simulink model "Simulink_7"  (R2013b)
settings: Solver=FixedStepDiscrete  StartTime=0.0  StopTime=100.0  FixedStep=1  RelTol=1e-3
undefined symbols (not defined in the file or in its folder): j, magnitude
settings Model: ExtModeAutoUpdateStatusClock=off  Creator=asteele  LastModifiedBy=99900361
settings DataIOCC: SignalLoggingSaveFormat=ModelDataLogs  SignalLoggingName=sigsOut
settings OptimizationCC: BooleanDataType=off
settings DebuggingCC: SaveWithParameterizedLinksMsg=none  SignalResolutionControl=TryResolveAllWithWarning  SolverPrmCheckMsg=none  MultiTaskDSMMsg=warning  MultiTaskCondExecSysMsg=none  StrictBusMsg=None
settings HardwareCC: TargetUnknown=on
settings RTWCC: IncludeERTFirstTime=on
settings GRTTargetCC: CombineOutputUpdateFcns=off  GRTInterface=on

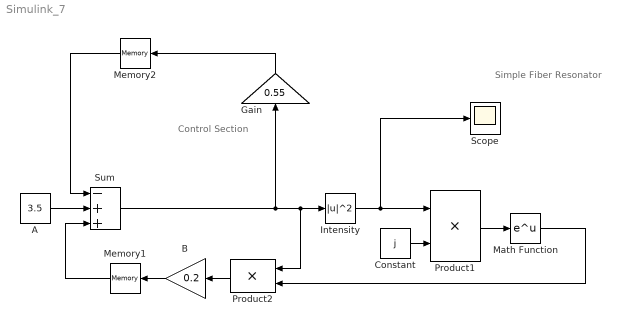
== system Simulink_7 ==
  note: Control Section
  note: Simple Fiber Resonator
  A : Constant  Value=3.5
  B : Gain  Gain=0.2  SaturateOnIntegerOverflow=on  OutDataTypeStr=Inherit: Same as input  ParamDataTypeStr=Inherit: Same as input
  Constant : Constant  Value=j
  Gain : Gain  Gain=0.55  SaturateOnIntegerOverflow=on  OutDataTypeStr=Inherit: Same as input  ParamDataTypeStr=Inherit: Same as input
  Intensity : Math  Operator=magnitude^2  SaturateOnIntegerOverflow=on
  Math Function : Math  SaturateOnIntegerOverflow=on
  Memory1 : Memory
  Memory2 : Memory
  Product1 : Product  SaturateOnIntegerOverflow=on  InputSameDT=on  OutDataTypeStr=Inherit: Same as first input
  Product2 : Product  SaturateOnIntegerOverflow=on  InputSameDT=on  OutDataTypeStr=Inherit: Same as first input
  Scope : Scope
      settings: TimeRange=400000
  Sum : Sum  Inputs=-++  SaturateOnIntegerOverflow=on  InputSameDT=on  OutDataTypeStr=Inherit: Same as first input
  wires:
  Intensity/1 -> Scope/1, Product1/1
  Product2/1 -> B/1
  B/1 -> Memory1/1
  Product1/1 -> Math Function/1
  Math Function/1 -> Product2/2
  Constant/1 -> Product1/2
  Gain/1 -> Memory2/1
  Memory1/1 -> Sum/3
  A/1 -> Sum/2
  Memory2/1 -> Sum/1
  Sum/1 -> Gain/1, Intensity/1, Product2/1
